simulink model "thermal_model"  (R2024b)
settings: Solver=VariableStepAuto  StartTime=0.0  StopTime=10.0  RelTol=1e-3
values from neighbouring files (symbols this model uses):
  C1 = 50    [task1.m]
  C2 = 60    [task1.m]
  qamp = 3    [task1.m]
  qtime = 10    [task1.m]
  R12 = (R1 * R2) / (R1 + R2)    (= 5)    [task1.m]
  R2 = 10    [task1.m]
  R23 = (R2 * R3) / (R2 + R3)    (= 5)    [task1.m]
settings Model: Creator=Rotim  LastModifiedBy=Rotim

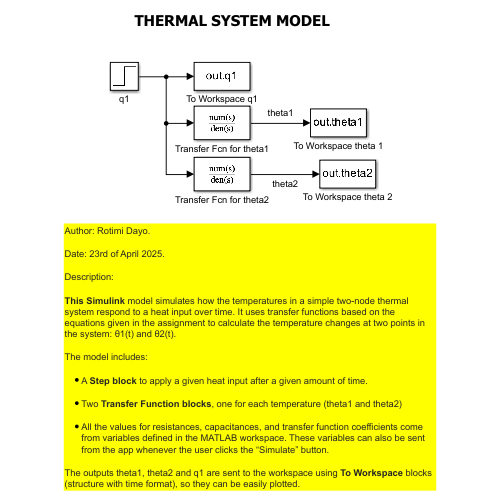
[thumbnail: Simulink's stored preview of the top-level diagram]
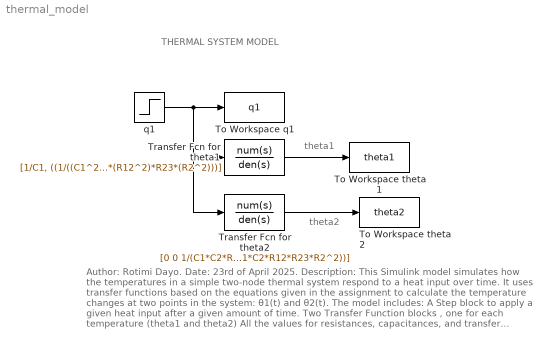
== system thermal_model ==
  note: theta2
  note: theta1
  note: Author: Rotimi Dayo.
      | Date: 23rd of April 2025.
      | Description:
      | This Simulink model simulates how the temperatures in a simple two-node thermal system respond to a heat input over time. It uses transfer functions based on the equations given in the assignment to calculate the temperature changes at two points in the system: θ1​(t) and θ2​(t).
      | The model includes:
      | A Step block to apply a given heat input after a given amount of time.
      | Two Transfer Function blocks , one for each temperature (theta1 and theta2)
      | All the values for resistances, capacitances, and transfer function coefficients come from variables defined in the MATLAB workspace. These variables can also be sent from the app whenever the user clicks the “Simulate” button.
      | The outputs theta1, theta2 and q1 are sent to the workspace using To Workspace blocks (structure with time format), so they can be easily plotted.
  note: THERMAL SYSTEM MODEL
  To Workspace q1 : ToWorkspace  VariableName=q1  SaveFormat=Structure With Time  SampleTime=-1
  To Workspace theta 1 : ToWorkspace  VariableName=theta1  SaveFormat=Structure With Time  SampleTime=-1
  To Workspace theta 2 : ToWorkspace  VariableName=theta2  SaveFormat=Structure With Time  SampleTime=-1
  Transfer Fcn for theta1 : TransferFcn  Numerator=[1/C1, ((1/((C1^2)*R12)) + (1/(C1*C2*R23))), (1/((C1^2)*C2*R12*R23))]  Denominator=[1, ((2/(C1*R12)) + (1/(C2*R23))), ((1/((C1^2)*(R12^2))) + (1/(C1*C2*R12*R23)) + (((R2^2) - R12*R23)/(C1*C2*R12*R23*(R2^2)))), ((R2^2 - R12*R23)/((C1^2)*C2*(R12^2)*R23*(R2^2)))]
  Transfer Fcn for theta2 : TransferFcn  Numerator=[0 0 1/(C1*C2*R2)]  Denominator=[1, ((1/(C1*R12)) + (1/(C2*R23))), (((R2^2) - R12*R23)/(C1*C2*R12*R23*R2^2))]
  q1 : Step  Time=qtime * 60  After=qamp  SampleTime=0
  wires:
  q1/1 -> Transfer Fcn for theta2/1, Transfer Fcn for theta1/1, To Workspace q1/1
  Transfer Fcn for theta2/1 -> To Workspace theta 2/1
  Transfer Fcn for theta1/1 -> To Workspace theta 1/1
